simulink model "Subsystem"  (R2020b)
settings: Solver=VariableStepAuto  StartTime=0.0  StopTime=10.0  RelTol=1e-3
settings Model: Creator=HP  LastModifiedBy=HP
settings DataIOCC: SaveOutput=off  SaveTime=off

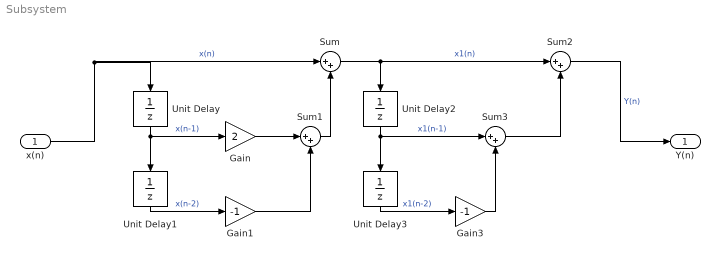
== system Subsystem ==
  x(n) : Inport  OutDataTypeStr=double  PortDimensions=1  SampleTime=0
  Gain : Gain  Gain=2
  Gain1 : Gain  Gain=-1
  Gain3 : Gain  Gain=-1
  Sum{,1..3} (4 alike) : Sum  Inputs=|++
  Unit Delay{,1..3} (4 alike) : UnitDelay  SampleTime=-1  HasFrameUpgradeWarning=on
  Y(n) : Outport  OutDataTypeStr=double  PortDimensions=1  SampleTime=0
  wires:
  x(n)/1 -> Unit Delay/1, Sum/1  "x(n)"
  Unit Delay/1 -> Gain/1, Unit Delay1/1  "x(n-1)"
  Sum1/1 -> Sum/2
  Sum2/1 -> Y(n)/1  "Y(n)"
  Gain1/1 -> Sum1/2
  Sum/1 -> Sum2/1, Unit Delay2/1  "x1(n)"
  Gain/1 -> Sum1/1
  Unit Delay1/1 -> Gain1/1  "x(n-2)"
  Gain3/1 -> Sum3/2
  Sum3/1 -> Sum2/2
  Unit Delay2/1 -> Unit Delay3/1, Sum3/1  "x1(n-1)"
  Unit Delay3/1 -> Gain3/1  "x1(n-2)"
